simulink model "BreakDownControll"  (R2022b)
settings: Solver=FixedStepDiscrete  StartTime=0.0  StopTime=10.0  RelTol=1e-3
undefined symbols (not defined in the file): KfBaseTimer_ms, KfBaseTimerV_ms, KfLowerTempthreshold_value, KfLowerVThreshold_mV, KfPWM_BaseTime_ms, KfPWM_OnDebTime_ms, KfPWM_PeriodTime_ms, KfTriggerTimer_ms, KfTriggerTimerV_ms, KfUpperTempThreshold_value, KfUpperVThreshold_mV, KuFailSafeOverRide_null, KuFailSafeSwitch_null
libraries: simulink x2
settings Model: DataDictionary=BreakDownControll.sldd  Creator=zhaoyu  LastModifiedBy=zhaoyu
settings OptimizationCC: DefaultParameterBehavior=Inlined  EnhancedBackFolding=on  PassReuseOutputArgsAs=Individual arguments  ZeroExternalMemoryAtStartup=off  ZeroInternalMemoryAtStartup=off  OptimizeBlockOrder=speed  DifferentSizesBufferReuse=on  OptimizationCustomize=off  EfficientTunableParamExpr=on
settings DebuggingCC: ParameterTunabilityLossMsg=error
settings SFSimCC: SimGenImportedTypeDefs=on  MATLABDynamicMemAlloc=off
settings RTWCC: Description=Embedded Coder  SystemTargetFile=ert.tlc  TemplateMakefile=ert_default_tmf
settings CodeAppCC: ForceParamTrailComments=on  IgnoreCustomStorageClasses=off  OperatorAnnotations=on  SimulinkDataObjDesc=on  SFDataObjDesc=on  InsertBlockDesc=on
settings ERTTargetCC: TargetLangStandard=C99 (ISO)  GenerateSampleERTMain=on  InlinedParameterPlacement=NonHierarchical  ERTCustomFileTemplate=example_file_process.tlc

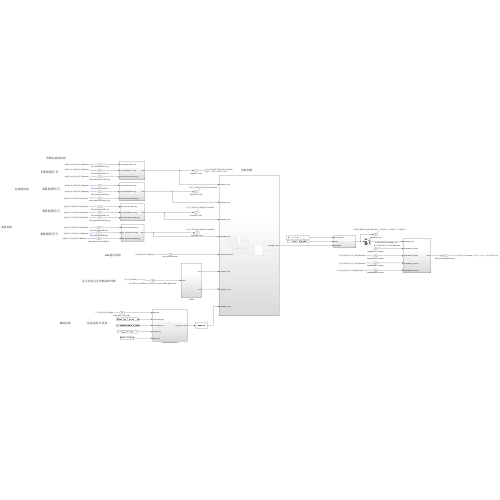
[thumbnail: Simulink's stored preview of the top-level diagram]
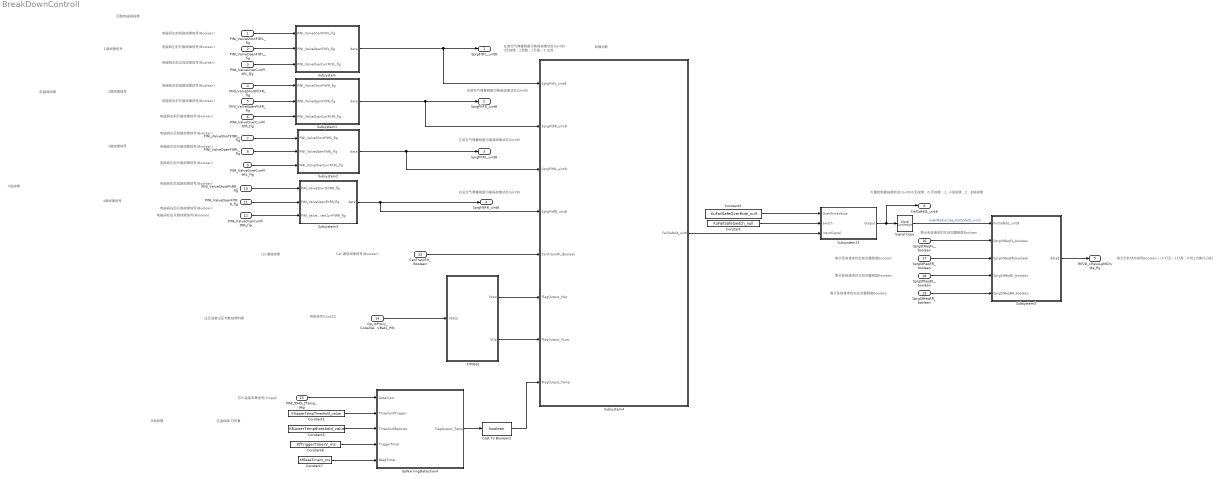
== system BreakDownControll ==
  note: 表示系统请求的左前空簧刚度Boolean
  note: 外置控制器故障状态(Uint8)0无故障；0:无故障；1：A级故障；2：B级故障
  note: 左前空气弹簧刚度切换阀故障状态(Uint8)
      | 0无故障；1短路；2开路；3 过流
  note: 芯片温度采集信号(Single)
  note: Can通信故障信号(Boolean)
  note: 电磁阀左前短路故障信号(Boolean)
  note: 故障判断
  note: 过压或者过压判断故障判断
  note: can通信故障
  note: 电磁阀故障
  note: A级故障
  note: 4路故障信号
  note: 四路电磁阀故障
  note: 1路故障信号
  note: 2路故障信号
  note: 过温故障,可恢复
  note: B级故障
  note: 3路故障信号
  note: 电磁阀左前开路故障信号(Boolean)
  note: 电磁阀左前过流故障信号(Boolean)
  note: 电磁阀右前短路故障信号(Boolean)
  note: 电磁阀右前开路故障信号(Boolean)
  note: 电磁阀右前开路故障信号(Boolean)
  note: 电磁阀左后短路故障信号(Boolean)
  note: 电磁阀左后开路故障信号(Boolean)
  note: 电磁阀左后开路故障信号(Boolean)
  note: 电磁阀右后短路故障信号(Boolean)
  note: 电磁阀右后开路故障信号(Boolean)
  note: 电磁阀右后开路故障信号(Boolean)
  note: 供电信号(Uint32)
  note: 右前空气弹簧刚度切换阀故障状态(Uint8)
  note: 左后空气弹簧刚度切换阀故障状态(Uint8)
  note: 右后空气弹簧刚度切换阀故障状态(Uint8)
  note: 表示系统请求的右前空簧刚度Boolean
  note: 表示系统请求的左后空簧刚度Boolean
  note: 表示系统请求的右后空簧刚度Boolean
  note: 表示灯的状态信号Boolean）(0 灯灭；1灯亮；0 和1切换灯闪烁)
  PINI_ValveShortFltFL_flg : Inport
  PINI_ValveOpenFltFL_flg : Inport  Port=2
  PINI_ValveOverCurrFltFL_flg : Inport  Port=3
  PINI_ValveShortFltFR_flg : Inport  Port=4
  PINI_ValveOpenFltFR_flg : Inport  Port=5
  PINI_ValveOverCurrFltFR_flg : Inport  Port=6
  PINI_ValveShortFltRL_flg : Inport  Port=7
  PINI_ValveOpenFltRL_flg : Inport  Port=8
  PINI_ValveOverCurrFltRL_flg : Inport  Port=9
  PINI_ValveShortFltRR_flg : Inport  Port=10
  PINI_ValveOpenFltRR_flg : Inport  Port=11
  PINI_ValveOverCurrFltRR_flg : Inport  Port=12
  CanTransFlt_Boolean : Inport  Port=13
  Gp_IoProxy_Core2Send_Gp_IoProxy_Core2_uVfPINI_VBat2_PIN : Inport  Port=14
  PINI_9945_2Temp_deg : Inport  Port=15
  SprgStReqFL_boolean : Inport  Port=16
  SprgStReqFR_boolean : Inport  Port=17
  SprgStReqRL_boolean : Inport  Port=18
  SprgStReqRR_boolean : Inport  Port=19
  Cast To Boolean2 : DataTypeConversion  OutDataTypeStr=boolean  SaturateOnIntegerOverflow=off  RndMeth=Floor
  Constant : Constant  Value=KuFailSafeSwitch_null
  Constant1 : Constant  Value=KfUpperTempThreshold_value  OutDataTypeStr=single
  Constant2 : Constant  Value=KuFailSafeOverRide_null
  Constant5 : Constant  Value=KfLowerTempthreshold_value  OutDataTypeStr=single
  Constant6 : Constant  Value=KfTriggerTimerV_ms  OutDataTypeStr=single
  Constant7 : Constant  Value=KfBaseTimerV_ms  OutDataTypeStr=single
  FltVBat : Subsystem
  Signal Copy : SignalConversion  OverrideOpt=off
  Subsystem : Subsystem
  Subsystem1 : Subsystem
  Subsystem2 : Subsystem
  Subsystem23 : Subsystem
  Subsystem3 : Subsystem
  Subsystem4 : Subsystem
  Subsystem5 : Subsystem
  UpWarningDetectionA : Subsystem
  SprgFltFL_uint8 : Outport
  SprgFltFR_uint8 : Outport  Port=2
  SprgFltRL_uint8 : Outport  Port=3
  SprgFltRR_uint8 : Outport  Port=4
  REVD_LRevsLghtDrvSts_flg : Outport  Port=5
  FailSafeSt_uint8 : Outport  Port=6  OutDataTypeStr=uint8
  wires:
  UpWarningDetectionA/1(FlagOutput_Temp) -> Cast To Boolean2/1
  Constant2/1 -> Subsystem23/1(OverWriteValue)
  PINI_ValveShortFltFR_flg/1 -> Subsystem1/1(PINI_ValveShortFltFR_flg)
  PINI_ValveShortFltRR_flg/1 -> Subsystem3/1(PINI_ValveShortFltRR_flg)
  Gp_IoProxy_Core2Send_Gp_IoProxy_Core2_uVfPINI_VBat2_PIN/1 -> FltVBat/1(Vbat2)
  Signal Copy/1 -> Subsystem5/1(FailSafeSt_uint8)  "VuAirRadiotube_FailSafeSt_nul1l"
  PINI_ValveOverCurrFltRR_flg/1 -> Subsystem3/3(PINI_ValveOverCurrFltRR_flg)
  FltVBat/2(VUp) -> Subsystem4/7(FlagOutput_VLow)
  FltVBat/1(VLow) -> Subsystem4/6(FlagOutput_VUp)
  PINI_ValveOverCurrFltFR_flg/1 -> Subsystem1/3(PINI_ValveOverCurrFltFR_flg)
  Subsystem2/1(data) -> Subsystem4/3(SprgFltRL_uint8), SprgFltRL_uint8/1
  Cast To Boolean2/1 -> Subsystem4/8(FlagOutput_Temp)
  SprgStReqRR_boolean/1 -> Subsystem5/5(SprgStReqRR_boolean)
  Constant7/1 -> UpWarningDetectionA/5(BaseTimer)
  Constant6/1 -> UpWarningDetectionA/4(TriggerTimer)
  Subsystem1/1(data) -> Subsystem4/2(SprgFltFR_uint8), SprgFltFR_uint8/1
  SprgStReqFL_boolean/1 -> Subsystem5/2(SprgStReqFL_boolean)
  CanTransFlt_Boolean/1 -> Subsystem4/5(CanTransFlt_Boolean)
  Subsystem4/1(FailSafeSt_uint8) -> Subsystem23/3(inputSignal)
  PINI_ValveOpenFltRR_flg/1 -> Subsystem3/2(PINI_ValveOpenFltRR_flg)
  Subsystem3/1(data) -> Subsystem4/4(SprgFltRR_uint8), SprgFltRR_uint8/1
  Constant5/1 -> UpWarningDetectionA/3(ThresholdRecover)
  Subsystem23/1(Output) -> FailSafeSt_uint8/1, Signal Copy/1
  PINI_ValveOverCurrFltRL_flg/1 -> Subsystem2/3(PINI_ValveOverCurrFltRL_flg)
  Constant/1 -> Subsystem23/2(switch)
  Subsystem/1(data) -> Subsystem4/1(SprgFltFL_uint8), SprgFltFL_uint8/1
  SprgStReqFR_boolean/1 -> Subsystem5/3(SprgStReqFR_boolean)
  PINI_ValveOpenFltRL_flg/1 -> Subsystem2/2(PINI_ValveOpenFltRL_flg)
  Subsystem5/1(data2) -> REVD_LRevsLghtDrvSts_flg/1
  PINI_ValveShortFltRL_flg/1 -> Subsystem2/1(PINI_ValveShortFltRL_flg)
  SprgStReqRL_boolean/1 -> Subsystem5/4(SprgStReqRL_boolean)
  PINI_ValveOverCurrFltFL_flg/1 -> Subsystem/3(PINI_ValveOverCurrFltFL_flg)
  PINI_ValveOpenFltFL_flg/1 -> Subsystem/2(PINI_ValveOpenFltFL_flg)
  Constant1/1 -> UpWarningDetectionA/2(ThresholdTrigger)
  PINI_ValveShortFltFL_flg/1 -> Subsystem/1(PINI_ValveShortFltFL_flg)
  PINI_ValveOpenFltFR_flg/1 -> Subsystem1/2(PINI_ValveOpenFltFR_flg)
  PINI_9945_2Temp_deg/1 -> UpWarningDetectionA/1(DataInput)

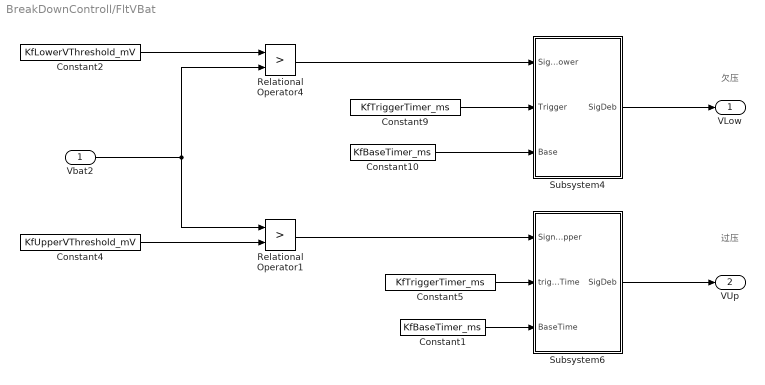
== system BreakDownControll/FltVBat ==
  note: 过压
  note: 欠压
  Vbat2 : Inport
  Constant1 : Constant  Value=KfBaseTimer_ms  OutDataTypeStr=Inherit: Inherit via back propagation
  Constant10 : Constant  Value=KfBaseTimer_ms  OutDataTypeStr=Inherit: Inherit via back propagation
  Constant2 : Constant  Value=KfLowerVThreshold_mV  VectorParams1D=off  OutDataTypeStr=uint32
  Constant4 : Constant  Value=KfUpperVThreshold_mV  VectorParams1D=off  OutDataTypeStr=uint32
  Constant5 : Constant  Value=KfTriggerTimer_ms  OutDataTypeStr=Inherit: Inherit via back propagation
  Constant9 : Constant  Value=KfTriggerTimer_ms  OutDataTypeStr=Inherit: Inherit via back propagation
  Relational Operator1 : RelationalOperator  Operator=>  OutDataTypeStr=boolean  RndMeth=Simplest  InputSameDT=off
  Relational Operator4 : RelationalOperator  Operator=>  OutDataTypeStr=boolean  RndMeth=Simplest  InputSameDT=off
  Subsystem4 : Subsystem
  Subsystem6 : Subsystem
  VLow : Outport  VectorParamsAs1DForOutWhenUnconnected=off
      settings: EnsureOutportIsVirtual=on
  VUp : Outport  Port=2  VectorParamsAs1DForOutWhenUnconnected=off
      settings: EnsureOutportIsVirtual=on
  wires:
  Constant10/1 -> Subsystem4/3(Base)
  Constant1/1 -> Subsystem6/3(BaseTime)
  Subsystem4/1(SigDeb) -> VLow/1
  Constant9/1 -> Subsystem4/2(Trigger)
  Constant5/1 -> Subsystem6/2(triggerTime)
  Constant4/1 -> Relational Operator1/2
  Relational Operator4/1 -> Subsystem4/1(SignalLower)
  Relational Operator1/1 -> Subsystem6/1(SignalUpper)
  Vbat2/1 -> Relational Operator4/2, Relational Operator1/1
  Subsystem6/1(SigDeb) -> VUp/1
  Constant2/1 -> Relational Operator4/1

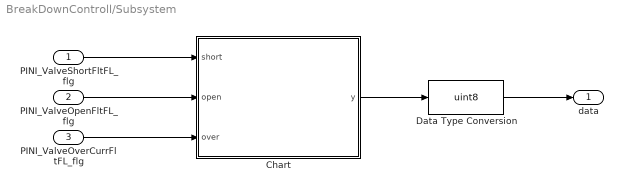
== system BreakDownControll/Subsystem ==
  PINI_ValveShortFltFL_flg : Inport
  PINI_ValveOpenFltFL_flg : Inport  Port=2
  PINI_ValveOverCurrFltFL_flg : Inport  Port=3
  Chart : Stateflow chart  TreatAsAtomicUnit=on
  Data Type Conversion : DataTypeConversion  OutDataTypeStr=uint8  SaturateOnIntegerOverflow=off  RndMeth=Floor
  data : Outport
  wires:
  PINI_ValveShortFltFL_flg/1 -> Chart/1(short)
  PINI_ValveOpenFltFL_flg/1 -> Chart/2(open)
  PINI_ValveOverCurrFltFL_flg/1 -> Chart/3(over)
  Chart/1(y) -> Data Type Conversion/1
  Data Type Conversion/1 -> data/1

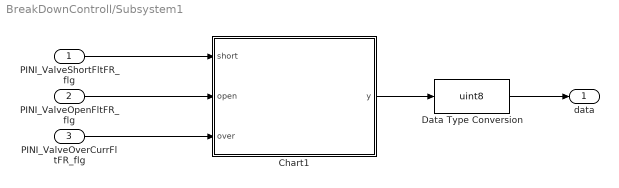
== system BreakDownControll/Subsystem1 ==
  PINI_ValveShortFltFR_flg : Inport
  PINI_ValveOpenFltFR_flg : Inport  Port=2
  PINI_ValveOverCurrFltFR_flg : Inport  Port=3
  Chart1 : Stateflow chart  TreatAsAtomicUnit=on
  Data Type Conversion : DataTypeConversion  OutDataTypeStr=uint8  SaturateOnIntegerOverflow=off  RndMeth=Floor
  data : Outport
  wires:
  PINI_ValveShortFltFR_flg/1 -> Chart1/1(short)
  PINI_ValveOpenFltFR_flg/1 -> Chart1/2(open)
  PINI_ValveOverCurrFltFR_flg/1 -> Chart1/3(over)
  Chart1/1(y) -> Data Type Conversion/1
  Data Type Conversion/1 -> data/1

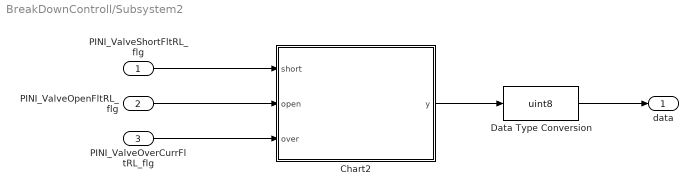
== system BreakDownControll/Subsystem2 ==
  PINI_ValveShortFltRL_flg : Inport
  PINI_ValveOpenFltRL_flg : Inport  Port=2
  PINI_ValveOverCurrFltRL_flg : Inport  Port=3
  Chart2 : Stateflow chart  TreatAsAtomicUnit=on
  Data Type Conversion : DataTypeConversion  OutDataTypeStr=uint8  SaturateOnIntegerOverflow=off  RndMeth=Floor
  data : Outport
  wires:
  PINI_ValveShortFltRL_flg/1 -> Chart2/1(short)
  PINI_ValveOpenFltRL_flg/1 -> Chart2/2(open)
  PINI_ValveOverCurrFltRL_flg/1 -> Chart2/3(over)
  Chart2/1(y) -> Data Type Conversion/1
  Data Type Conversion/1 -> data/1

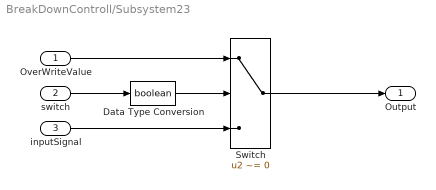
== system BreakDownControll/Subsystem23 ==
  OverWriteValue : Inport
  switch : Inport  Port=2
  inputSignal : Inport  Port=3
  Data Type Conversion : DataTypeConversion  OutDataTypeStr=boolean  SaturateOnIntegerOverflow=off  RndMeth=Floor
  Switch : Switch  Criteria=u2 ~= 0  SaturateOnIntegerOverflow=off  InputSameDT=off
  Output : Outport  VectorParamsAs1DForOutWhenUnconnected=off
  wires:
  Data Type Conversion/1 -> Switch/2
  Switch/1 -> Output/1
  switch/1 -> Data Type Conversion/1
  inputSignal/1 -> Switch/3
  OverWriteValue/1 -> Switch/1

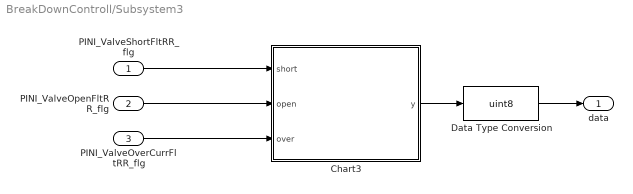
== system BreakDownControll/Subsystem3 ==
  PINI_ValveShortFltRR_flg : Inport
  PINI_ValveOpenFltRR_flg : Inport  Port=2
  PINI_ValveOverCurrFltRR_flg : Inport  Port=3
  Chart3 : Stateflow chart  TreatAsAtomicUnit=on
  Data Type Conversion : DataTypeConversion  OutDataTypeStr=uint8  SaturateOnIntegerOverflow=off  RndMeth=Floor
  data : Outport
  wires:
  PINI_ValveOverCurrFltRR_flg/1 -> Chart3/3(over)
  PINI_ValveOpenFltRR_flg/1 -> Chart3/2(open)
  PINI_ValveShortFltRR_flg/1 -> Chart3/1(short)
  Chart3/1(y) -> Data Type Conversion/1
  Data Type Conversion/1 -> data/1

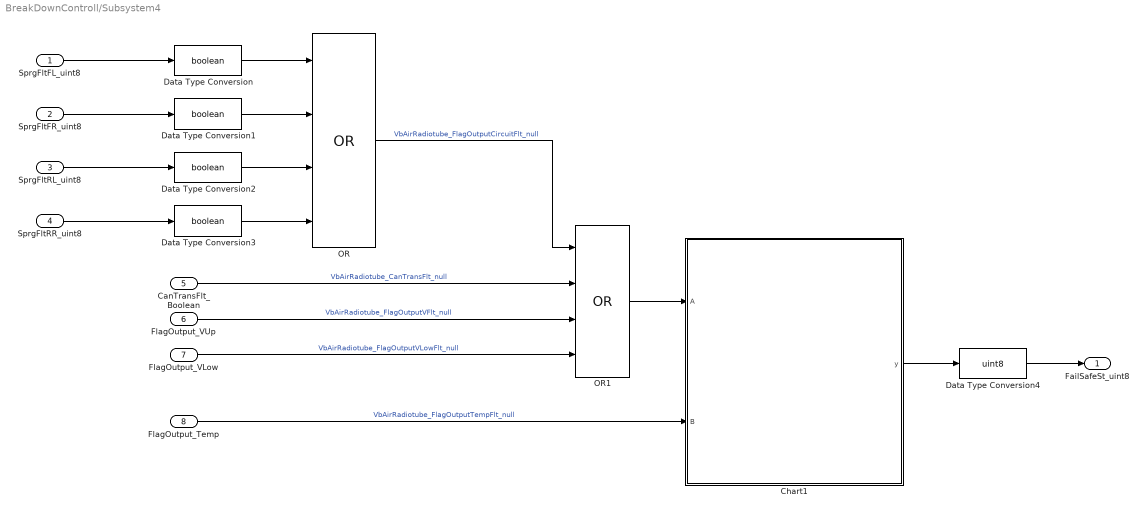
== system BreakDownControll/Subsystem4 ==
  SprgFltFL_uint8 : Inport
  SprgFltFR_uint8 : Inport  Port=2
  SprgFltRL_uint8 : Inport  Port=3
  SprgFltRR_uint8 : Inport  Port=4
  CanTransFlt_Boolean : Inport  Port=5
  FlagOutput_VUp : Inport  Port=6
  FlagOutput_VLow : Inport  Port=7
  FlagOutput_Temp : Inport  Port=8
  Chart1 : Stateflow chart  TreatAsAtomicUnit=on
  Data Type Conversion{,1..3} (4 alike) : DataTypeConversion  OutDataTypeStr=boolean  SaturateOnIntegerOverflow=off  RndMeth=Floor
  Data Type Conversion4 : DataTypeConversion  OutDataTypeStr=uint8  SaturateOnIntegerOverflow=off  RndMeth=Floor
  OR : Logic  Operator=OR  Inputs=4  AllPortsSameDT=off  OutDataTypeStr=boolean
  OR1 : Logic  Operator=OR  Inputs=4  AllPortsSameDT=off  OutDataTypeStr=boolean
  FailSafeSt_uint8 : Outport
  wires:
  SprgFltRR_uint8/1 -> Data Type Conversion3/1
  Data Type Conversion3/1 -> OR/4
  OR/1 -> OR1/1  "VbAirRadiotube_FlagOutputCircuitFlt_null"
  Data Type Conversion2/1 -> OR/3
  Data Type Conversion1/1 -> OR/2
  SprgFltFR_uint8/1 -> Data Type Conversion1/1
  Data Type Conversion/1 -> OR/1
  CanTransFlt_Boolean/1 -> OR1/2  "VbAirRadiotube_CanTransFlt_null"
  SprgFltFL_uint8/1 -> Data Type Conversion/1
  SprgFltRL_uint8/1 -> Data Type Conversion2/1
  FlagOutput_VUp/1 -> OR1/3  "VbAirRadiotube_FlagOutputVFlt_null"
  FlagOutput_Temp/1 -> Chart1/2(B)  "VbAirRadiotube_FlagOutputTempFlt_null"
  OR1/1 -> Chart1/1(A)
  Data Type Conversion4/1 -> FailSafeSt_uint8/1
  FlagOutput_VLow/1 -> OR1/4  "VbAirRadiotube_FlagOutputVLowFlt_null"
  Chart1/1(y) -> Data Type Conversion4/1

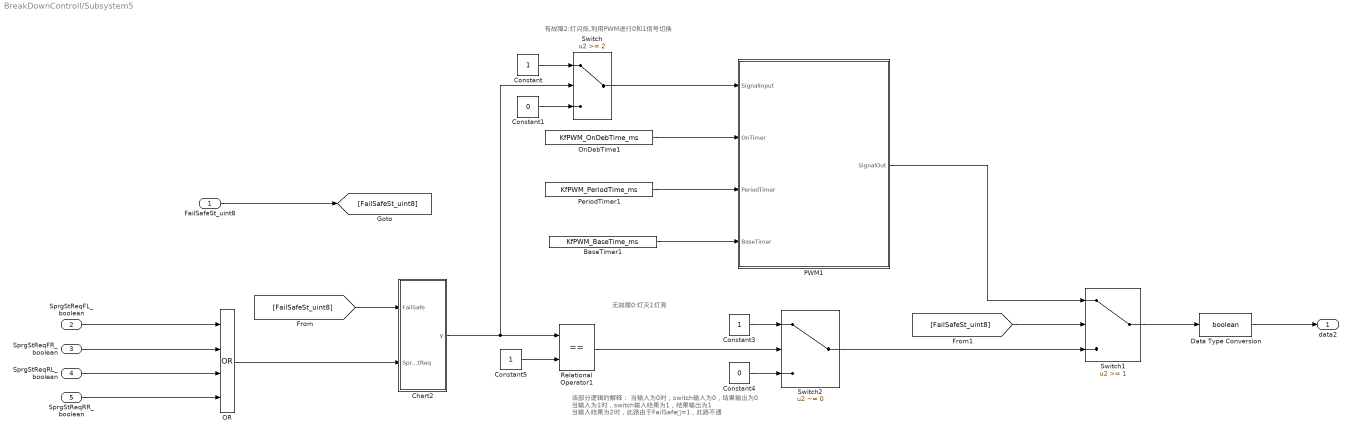
== system BreakDownControll/Subsystem5 ==
  note: 该部分逻辑的解释：
      | 当输入为0时，switch输入为0，结果输出为0
      | 当输入为1时，switch输入结果为1，结果输出为1
      | 当输入结果为2时，此路由于FailSafe〉=1，此路不通
  note: 有故障2:灯闪烁,利用PWM进行0和1信号切换
  note: 无故障0:灯灭1灯亮
  FailSafeSt_uint8 : Inport
  SprgStReqFL_boolean : Inport  Port=2
  SprgStReqFR_boolean : Inport  Port=3
  SprgStReqRL_boolean : Inport  Port=4
  SprgStReqRR_boolean : Inport  Port=5
  BaseTimer1 : Constant  Value=KfPWM_BaseTime_ms
  Chart2 : Stateflow chart  TreatAsAtomicUnit=on
  Constant : Constant
  Constant1 : Constant  Value=0
  Constant3 : Constant
  Constant4 : Constant  Value=0
  Constant5 : Constant
  Data Type Conversion : DataTypeConversion  OutDataTypeStr=boolean  SaturateOnIntegerOverflow=off  RndMeth=Floor
  OR : Logic  Operator=OR  Inputs=4  AllPortsSameDT=off  OutDataTypeStr=boolean
  OnDebTime1 : Constant  Value=KfPWM_OnDebTime_ms
  PWM1 : Subsystem
  PeriodTimer1 : Constant  Value=KfPWM_PeriodTime_ms
  Relational Operator1 : RelationalOperator  Operator===  OutDataTypeStr=boolean  RndMeth=Simplest  InputSameDT=off
  Switch : Switch  Threshold=2  SaturateOnIntegerOverflow=off  InputSameDT=off
  Switch1 : Switch  Threshold=1  OutDataTypeStr=boolean  SaturateOnIntegerOverflow=off  InputSameDT=off
  Switch2 : Switch  Criteria=u2 ~= 0  Threshold=1  SaturateOnIntegerOverflow=off  InputSameDT=off
  data2 : Outport
  wires:
  SprgStReqRL_boolean/1 -> OR/3
  SprgStReqFR_boolean/1 -> OR/2
  SprgStReqRR_boolean/1 -> OR/4
  SprgStReqFL_boolean/1 -> OR/1
  OR/1 -> Chart2/2(SprgStReq)
  Switch1/1 -> Data Type Conversion/1
  FailSafeSt_uint8/1 -> [FailSafeSt_uint8]
  [FailSafeSt_uint8] -> Chart2/1(FailSafe)
  Data Type Conversion/1 -> data2/1
  [FailSafeSt_uint8] -> Switch1/2
  Constant1/1 -> Switch/3
  Constant/1 -> Switch/1
  Switch/1 -> PWM1/1(SignalInput)
  Chart2/1(y) -> Relational Operator1/1, Switch/2
  PeriodTimer1/1 -> PWM1/3(PeriodTimer)
  BaseTimer1/1 -> PWM1/4(BaseTimer)
  OnDebTime1/1 -> PWM1/2(OnTimer)
  PWM1/1(SignalOut) -> Switch1/1
  Relational Operator1/1 -> Switch2/2
  Constant3/1 -> Switch2/1
  Switch2/1 -> Switch1/3
  Constant4/1 -> Switch2/3
  Constant5/1 -> Relational Operator1/2

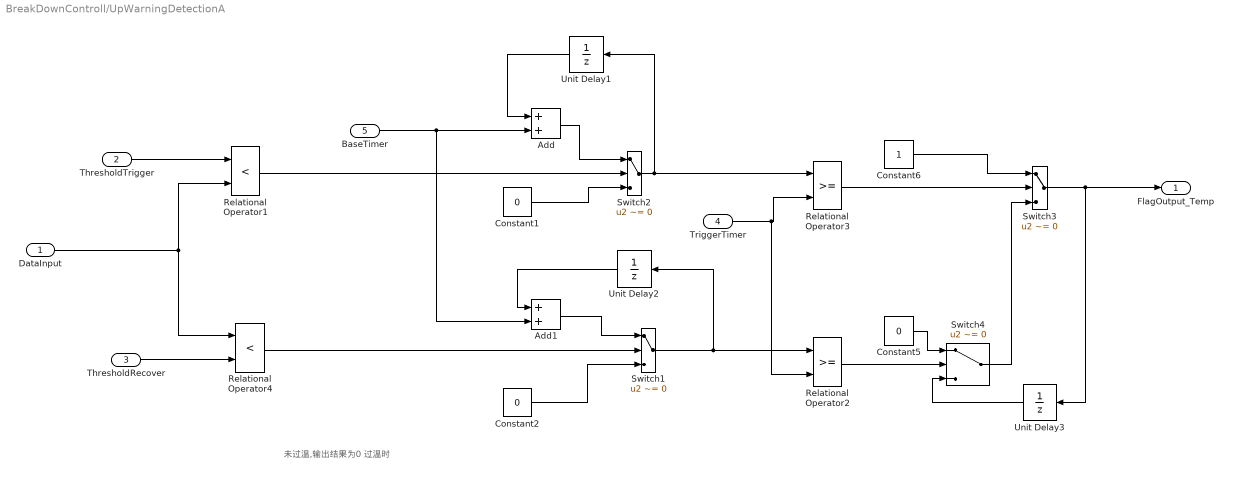
== system BreakDownControll/UpWarningDetectionA ==
  note: 未过温,输出结果为0
      | 过温时
  DataInput : Inport
  ThresholdTrigger : Inport  Port=2
  ThresholdRecover : Inport  Port=3
  TriggerTimer : Inport  Port=4
  BaseTimer : Inport  Port=5
  Add : Sum  InputSameDT=on  RndMeth=Round  SaturateOnIntegerOverflow=on  OutDataTypeStr=Inherit: Same as first input
  Add1 : Sum  InputSameDT=on  RndMeth=Round  SaturateOnIntegerOverflow=on  OutDataTypeStr=Inherit: Same as first input
  Constant1 : Constant  Value=0  OutDataTypeStr=Inherit: Inherit via back propagation
  Constant2 : Constant  Value=0  OutDataTypeStr=Inherit: Inherit via back propagation
  Constant5 : Constant  Value=0  OutDataTypeStr=uint8
  Constant6 : Constant  OutDataTypeStr=uint8
  Relational Operator1 : RelationalOperator  Operator=<  OutDataTypeStr=fixdt(0,8)
  Relational Operator2 : RelationalOperator  OutDataTypeStr=fixdt(0,8)
  Relational Operator3 : RelationalOperator  OutDataTypeStr=fixdt(0,8)
  Relational Operator4 : RelationalOperator  Operator=<  OutDataTypeStr=fixdt(0,8)
  Switch{1..4} (4 alike) : Switch  Criteria=u2 ~= 0  Threshold=1  OutDataTypeStr=Inherit: Inherit via back propagation  RndMeth=Round
      settings: AttributesFormatString=%<Criteria>
  Unit Delay1 : UnitDelay  SampleTime=-1  HasFrameUpgradeWarning=on
      settings: AttributesFormatString=Initial Value=%<InitialCondition>
  Unit Delay2 : UnitDelay  SampleTime=-1  HasFrameUpgradeWarning=on
      settings: AttributesFormatString=Initial Value=%<InitialCondition>
  Unit Delay3 : UnitDelay  SampleTime=-1  HasFrameUpgradeWarning=on
      settings: AttributesFormatString=Initial Value=%<InitialCondition>
  FlagOutput_Temp : Outport
  wires:
  Relational Operator2/1 -> Switch4/2
  BaseTimer/1 -> Add1/2, Add/2
  Switch2/1 -> Relational Operator3/1, Unit Delay1/1
  Relational Operator3/1 -> Switch3/2
  Add1/1 -> Switch1/1
  Relational Operator4/1 -> Switch1/2
  Constant1/1 -> Switch2/3
  Relational Operator1/1 -> Switch2/2
  Unit Delay1/1 -> Add/1
  ThresholdTrigger/1 -> Relational Operator1/1
  Unit Delay2/1 -> Add1/1
  Switch3/1 -> Unit Delay3/1, FlagOutput_Temp/1
  Switch4/1 -> Switch3/3
  ThresholdRecover/1 -> Relational Operator4/2
  DataInput/1 -> Relational Operator1/2, Relational Operator4/1
  Add/1 -> Switch2/1
  Switch1/1 -> Relational Operator2/1, Unit Delay2/1
  Unit Delay3/1 -> Switch4/3
  Constant5/1 -> Switch4/1
  TriggerTimer/1 -> Relational Operator2/2, Relational Operator3/2
  Constant2/1 -> Switch1/3
  Constant6/1 -> Switch3/1

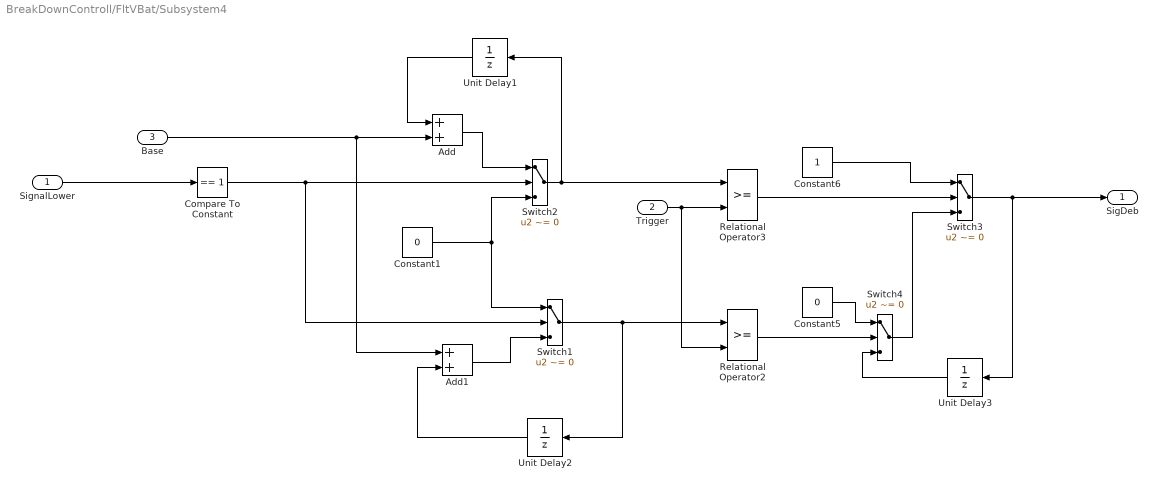
== system BreakDownControll/FltVBat/Subsystem4 ==
  SignalLower : Inport
  Trigger : Inport  Port=2
  Base : Inport  Port=3
  Add : Sum  InputSameDT=on  RndMeth=Round  SaturateOnIntegerOverflow=on  OutDataTypeStr=Inherit: Same as first input
  Add1 : Sum  InputSameDT=on  RndMeth=Round  SaturateOnIntegerOverflow=on  OutDataTypeStr=Inherit: Same as first input
  Compare To Constant : simulink/Logic and Bit Operations/Compare To Constant  relop===  const=1  OutDataTypeStr=uint8
  Constant1 : Constant  Value=0  OutDataTypeStr=Inherit: Inherit via back propagation
  Constant5 : Constant  Value=0  OutDataTypeStr=boolean
  Constant6 : Constant  OutDataTypeStr=boolean
  Relational Operator2 : RelationalOperator  OutDataTypeStr=fixdt(0,8)
  Relational Operator3 : RelationalOperator  OutDataTypeStr=fixdt(0,8)
  Switch{1..4} (4 alike) : Switch  Criteria=u2 ~= 0  Threshold=1  OutDataTypeStr=Inherit: Inherit via back propagation  RndMeth=Round
      settings: AttributesFormatString=%<Criteria>
  Unit Delay1 : UnitDelay  SampleTime=-1  HasFrameUpgradeWarning=on
      settings: AttributesFormatString=Initial Value=%<InitialCondition>
  Unit Delay2 : UnitDelay  SampleTime=-1  HasFrameUpgradeWarning=on
      settings: AttributesFormatString=Initial Value=%<InitialCondition>
  Unit Delay3 : UnitDelay  SampleTime=-1  HasFrameUpgradeWarning=on
      settings: AttributesFormatString=Initial Value=%<InitialCondition>
  SigDeb : Outport
  wires:
  Trigger/1 -> Relational Operator2/2, Relational Operator3/2
  SignalLower/1 -> Compare To Constant/1
  Base/1 -> Add1/1, Add/2
  Compare To Constant/1 -> Switch1/2, Switch2/2
  Add/1 -> Switch2/1
  Unit Delay2/1 -> Add1/2
  Switch4/1 -> Switch3/3
  Unit Delay1/1 -> Add/1
  Constant5/1 -> Switch4/1
  Switch3/1 -> SigDeb/1, Unit Delay3/1
  Relational Operator3/1 -> Switch3/2
  Switch1/1 -> Relational Operator2/1, Unit Delay2/1
  Constant1/1 -> Switch2/3, Switch1/1
  Switch2/1 -> Relational Operator3/1, Unit Delay1/1
  Add1/1 -> Switch1/3
  Unit Delay3/1 -> Switch4/3
  Relational Operator2/1 -> Switch4/2
  Constant6/1 -> Switch3/1

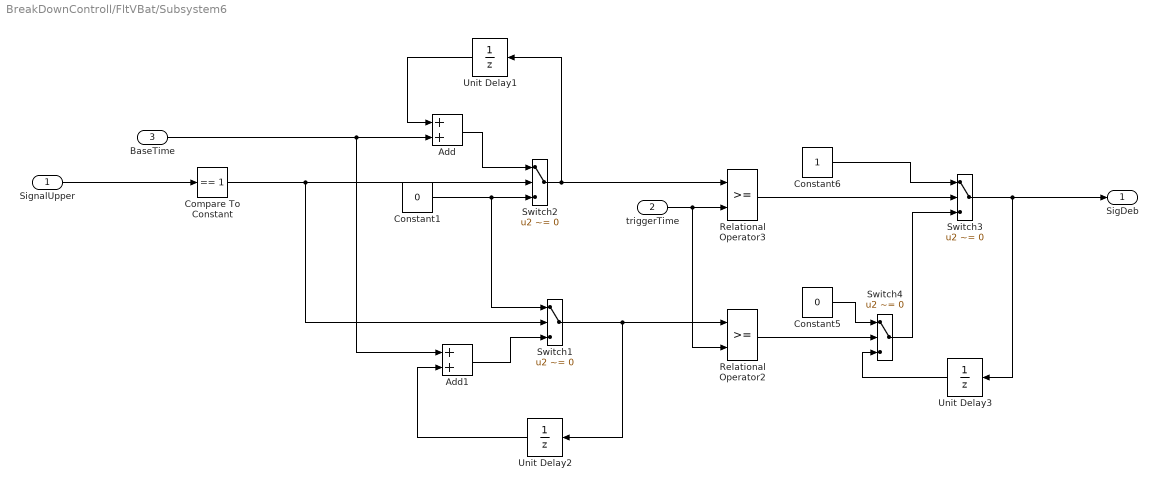
== system BreakDownControll/FltVBat/Subsystem6 ==
  SignalUpper : Inport
  triggerTime : Inport  Port=2
  BaseTime : Inport  Port=3
  Add : Sum  InputSameDT=on  RndMeth=Round  SaturateOnIntegerOverflow=on  OutDataTypeStr=Inherit: Same as first input
  Add1 : Sum  InputSameDT=on  RndMeth=Round  SaturateOnIntegerOverflow=on  OutDataTypeStr=Inherit: Same as first input
  Compare To Constant : simulink/Logic and Bit Operations/Compare To Constant  relop===  const=1  OutDataTypeStr=uint8
  Constant1 : Constant  Value=0  OutDataTypeStr=Inherit: Inherit via back propagation
  Constant5 : Constant  Value=0  OutDataTypeStr=boolean
  Constant6 : Constant  OutDataTypeStr=boolean
  Relational Operator2 : RelationalOperator  OutDataTypeStr=fixdt(0,8)
  Relational Operator3 : RelationalOperator  OutDataTypeStr=fixdt(0,8)
  Switch{1..4} (4 alike) : Switch  Criteria=u2 ~= 0  Threshold=1  OutDataTypeStr=Inherit: Inherit via back propagation  RndMeth=Round
      settings: AttributesFormatString=%<Criteria>
  Unit Delay1 : UnitDelay  SampleTime=-1  HasFrameUpgradeWarning=on
      settings: AttributesFormatString=Initial Value=%<InitialCondition>
  Unit Delay2 : UnitDelay  SampleTime=-1  HasFrameUpgradeWarning=on
      settings: AttributesFormatString=Initial Value=%<InitialCondition>
  Unit Delay3 : UnitDelay  SampleTime=-1  HasFrameUpgradeWarning=on
      settings: AttributesFormatString=Initial Value=%<InitialCondition>
  SigDeb : Outport
  wires:
  Constant6/1 -> Switch3/1
  Relational Operator2/1 -> Switch4/2
  Unit Delay3/1 -> Switch4/3
  Add1/1 -> Switch1/3
  Switch2/1 -> Unit Delay1/1, Relational Operator3/1
  Constant1/1 -> Switch2/3, Switch1/1
  Switch1/1 -> Unit Delay2/1, Relational Operator2/1
  Relational Operator3/1 -> Switch3/2
  Switch3/1 -> Unit Delay3/1, SigDeb/1
  Constant5/1 -> Switch4/1
  Unit Delay1/1 -> Add/1
  Switch4/1 -> Switch3/3
  Unit Delay2/1 -> Add1/2
  Add/1 -> Switch2/1
  Compare To Constant/1 -> Switch2/2, Switch1/2
  BaseTime/1 -> Add/2, Add1/1
  SignalUpper/1 -> Compare To Constant/1
  triggerTime/1 -> Relational Operator2/2, Relational Operator3/2

== system BreakDownControll/Subsystem5/PWM1 ==
  SignalInput : Inport
  OnTimer : Inport  Port=2
  PeriodTimer : Inport  Port=3
  BaseTimer : Inport  Port=4
  Chart : Stateflow chart  TreatAsAtomicUnit=on
  SignalOut : Outport
  wires:
  PeriodTimer/1 -> Chart/3(PeriodTimer)
  OnTimer/1 -> Chart/2(OnTimer)
  BaseTimer/1 -> Chart/4(BaseTimer)
  Chart/1(SignalOut) -> SignalOut/1
  SignalInput/1 -> Chart/1(SignalInput)

== stateflow chart BreakDownControll/Subsystem2/Chart2 ==
  (default) -> (junction 36) : % 0无故障；1短路；2开路；3。过流
  (junction 36) -> (junction 37) [order 1] : [short == 0 && open ==0 && over ==0]
  (junction 36) -> (junction 38) [order 2]
  (junction 37) -> (junction 45) : {y=0;}
  (junction 38) -> (junction 39) [order 1] : [short == 1 && open ==0 && over ==0]
  (junction 38) -> (junction 40) [order 2]
  (junction 39) -> (junction 44) : {y=1;}
  (junction 40) -> (junction 41) [order 1] : [short == 0 && open ==1 && over ==0]
  (junction 40) -> (junction 42) [order 2] : {y=3;}
  (junction 41) -> (junction 43) : {y=2;}
  (junction 43) -> (junction 42)
  (junction 44) -> (junction 43)
  (junction 45) -> (junction 44)
  (junction 42) -> (junction 46)
  data: short input; open input; over input; y output

== stateflow chart BreakDownControll/Subsystem3/Chart3 ==
  (default) -> (junction 36) : % 0无故障；1短路；2开路；3。过流
  (junction 36) -> (junction 37) [order 1] : [short == 0 && open ==0 && over ==0]
  (junction 36) -> (junction 38) [order 2]
  (junction 37) -> (junction 45) : {y=0;}
  (junction 38) -> (junction 39) [order 1] : [short == 1 && open ==0 && over ==0]
  (junction 38) -> (junction 40) [order 2]
  (junction 39) -> (junction 44) : {y=1;}
  (junction 40) -> (junction 41) [order 1] : [short == 0 && open ==1 && over ==0]
  (junction 40) -> (junction 42) [order 2] : {y=3;}
  (junction 41) -> (junction 43) : {y=2;}
  (junction 43) -> (junction 42)
  (junction 44) -> (junction 43)
  (junction 45) -> (junction 44)
  (junction 42) -> (junction 46)
  data: short input; open input; over input; y output

== stateflow chart BreakDownControll/Subsystem5/PWM1/Chart ==
  settings: executeAtInitialization=1
  state Init
    en:
    on_time_cnt=0;
    off_time_cnt=0;
    SignalOut=0;
  state count
    en:
    SignalOut=1;
    off_time_cnt=0;
    on_time_cnt=0;
    on_time_cnt=on_time_cnt+BaseTimer;
    du:
    on_time_cnt=on_time_cnt+BaseTimer;
  state OFF
    en:
    SignalOut=1;
    off_time_cnt=0;
    on_time_cnt=0;
    on_time_cnt=on_time_cnt+BaseTimer;
    du:
    on_time_cnt=on_time_cnt+BaseTimer;
  state ON
    en:
    SignalOut=0;
    off_time_cnt=0;
    on_time_cnt=0;
    off_time_cnt=off_time_cnt+BaseTimer;
    du:
    off_time_cnt=off_time_cnt+BaseTimer;
  (default) -> Init
  Init -> count : [SignalInput~=0]
  count -> Init [order 1] : [SignalInput==0]
  ON -> Init [order 2] : [SignalInput==0]
  count -> ON [order 2] : [on_time_cnt>=OnTimer]
  OFF -> Init [order 2] : [SignalInput==0]
  OFF -> ON [order 1] : [on_time_cnt>=OnTimer]
  ON -> OFF [order 1] : [off_time_cnt>=(PeriodTimer-OnTimer)]
  data: SignalOut output; on_time_cnt local; off_time_cnt local; SignalInput input; OnTimer input; PeriodTimer input; BaseTimer input

== stateflow chart BreakDownControll/Subsystem4/Chart1 ==
  (default) -> (junction 13) : % ０无故障；１Ａ级故障；２Ｂ级故障
  (junction 13) -> (junction 14) [order 1] : [A==1]
  (junction 13) -> (junction 15) [order 2]
  (junction 14) -> (junction 19) : {y=1;}
  (junction 15) -> (junction 16) [order 1] : [A== 0&& B ==1]
  (junction 15) -> (junction 17) [order 2] : {y=0;}
  (junction 16) -> (junction 18) : {y=2;}
  (junction 18) -> (junction 17)
  (junction 19) -> (junction 18)
  (junction 17) -> (junction 20)
  data: A input; y output; B input

== stateflow chart BreakDownControll/Subsystem5/Chart2 ==
  (default) -> (junction 42) : % %y=0代表低刚度,灯灭；y=1代表至少一个高刚度，灯亮；y=2代表故障 灯闪烁
      | % 输入的变量为刚度切换请求输入
  (junction 42) -> (junction 43) [order 1] : [FailSafe~=0 ]
  (junction 42) -> (junction 44) [order 2]
  (junction 43) -> (junction 48) : {y=2;}
  (junction 44) -> (junction 45) [order 1] : [FailSafe==0 && SprgStReq ==1]
  (junction 44) -> (junction 46) [order 2] : {y=0;}
  (junction 45) -> (junction 47) : {y=1;}
  (junction 47) -> (junction 46)
  (junction 48) -> (junction 47)
  (junction 46) -> (junction 49)
  data: FailSafe input; SprgStReq input; y output

== stateflow chart BreakDownControll/Subsystem/Chart ==
  (default) -> (junction 36) : % 0无故障；1短路；2开路；3 过流
  (junction 36) -> (junction 37) [order 1] : [short == 0 && open ==0 && over ==0]
  (junction 36) -> (junction 38) [order 2]
  (junction 37) -> (junction 45) : {y=0;}
  (junction 38) -> (junction 39) [order 1] : [short == 1 && open ==0 && over ==0]
  (junction 38) -> (junction 40) [order 2]
  (junction 39) -> (junction 44) : {y=1;}
  (junction 40) -> (junction 41) [order 1] : [short == 0 && open ==1 && over ==0]
  (junction 40) -> (junction 42) [order 2] : {y=3;}
  (junction 41) -> (junction 43) : {y=2;}
  (junction 43) -> (junction 42)
  (junction 44) -> (junction 43)
  (junction 45) -> (junction 44)
  (junction 42) -> (junction 46)
  data: short input; open input; over input; y output

== stateflow chart BreakDownControll/Subsystem1/Chart1 ==
  (default) -> (junction 36) : % 0无故障；1短路；2开路；3。过流
  (junction 36) -> (junction 37) [order 1] : [short == 0 && open ==0 && over ==0]
  (junction 36) -> (junction 38) [order 2]
  (junction 37) -> (junction 45) : {y=0;}
  (junction 38) -> (junction 39) [order 1] : [short == 1 && open ==0 && over ==0]
  (junction 38) -> (junction 40) [order 2]
  (junction 39) -> (junction 44) : {y=1;}
  (junction 40) -> (junction 41) [order 1] : [short == 0 && open ==1 && over ==0]
  (junction 40) -> (junction 42) [order 2] : {y=3;}
  (junction 41) -> (junction 43) : {y=2;}
  (junction 43) -> (junction 42)
  (junction 44) -> (junction 43)
  (junction 45) -> (junction 44)
  (junction 42) -> (junction 46)
  data: short input; open input; over input; y output
